simulink model "imageStreamKeyboard"  (Simulink 10.0)
settings: Solver=VariableStepDiscrete  StartTime=0.0  StopTime=1000.0  FixedStep=0.1  RelTol=1e-3  EnableMultiTasking=on
libraries: LemmingToolbox x6
settings Model: Creator=langmo  LastModifiedBy=unknown
settings DataIOCC: LimitDataPoints=on  SignalLoggingSaveFormat=ModelDataLogs
settings OptimizationCC: ExpressionDepthLimit=2147483647  InitFltsAndDblsToZero=on
settings DebuggingCC: SolverPrmCheckMsg=warning  FcnCallInpInsideContextMsg=warning  StateNameClashWarn=warning
settings SFSimCC: SimUseLocalCustomCode=on  CustomCodeUndefinedFunction=FilterOut
settings RTWCC: RTWUseLocalCustomCode=on

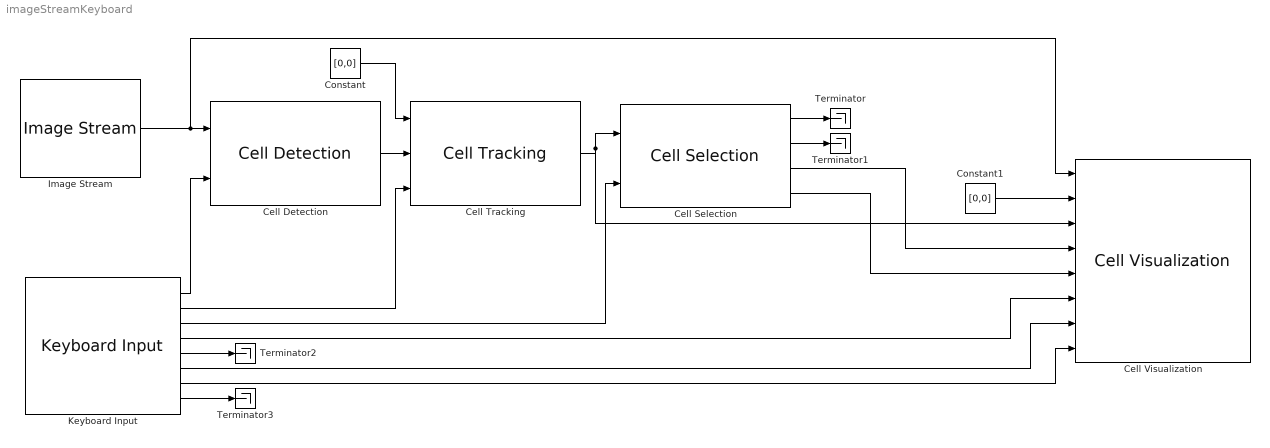
== system imageStreamKeyboard ==
  Cell Detection : LemmingToolbox/Cell Detection  SystemSampleTime=-1  imageDim=[1344,1024]  binning=2  cellSizeLowerLimit=70  cellSizeUpperLimit=2000  maxNumCells=1000  resizeScale=0.5  sampleTimes=[0.2, 0.1]
  Cell Selection : LemmingToolbox/Cell Selection  SystemSampleTime=-1  numFrames=8  maxNumCells=1000  sampleTimes=[0.2, 0.1]
  Cell Tracking : LemmingToolbox/Cell Tracking  SystemSampleTime=-1  maxDistance=0.1  maxNumCells=1000  tKeepLost=10  sampleTimes=[0.2, 0.1]
  Cell Visualization : LemmingToolbox/Cell Visualization  SystemSampleTime=-1  outputFilename=simulation.avi  imageDim=[1344,1024]  binning=2  maxNumCells=1000  coneWidth=150  coneAngle=pi/4  pathLength=30  sampleTimes=[0.3, 0.1]
  Constant : Constant  Value=[0,0]
  Constant1 : Constant  Value=[0,0]
  Image Stream : LemmingToolbox/Image Stream  SystemSampleTime=-1  imageDir=matlabroot/toolbox/LemmingToolbox/dummyImages  binning=2  sampleTimes=[0.2,0.1]
  Keyboard Input : LemmingToolbox/Keyboard Input  SystemSampleTime=1  initThreshold=0.015  sampleTimes=[0.2, 0.1]
  Terminator{,1..3} (4 alike) : Terminator
  wires:
  Image Stream/1 -> Cell Detection/1, Cell Visualization/1
  Cell Selection/3 -> Cell Visualization/4
  Cell Tracking/1 -> Cell Selection/1, Cell Visualization/3
  Keyboard Input/1 -> Cell Detection/2
  Keyboard Input/3 -> Cell Selection/2
  Cell Detection/1 -> Cell Tracking/2
  Keyboard Input/2 -> Cell Tracking/3
  Cell Selection/4 -> Cell Visualization/5
  Keyboard Input/4 -> Cell Visualization/6
  Keyboard Input/6 -> Cell Visualization/7
  Keyboard Input/7 -> Cell Visualization/8
  Constant/1 -> Cell Tracking/1
  Constant1/1 -> Cell Visualization/2
  Cell Selection/1 -> Terminator/1
  Cell Selection/2 -> Terminator1/1
  Keyboard Input/5 -> Terminator2/1
  Keyboard Input/8 -> Terminator3/1
